simulink model "window_design"  (R2012b)
settings: Solver=ode45  StartTime=0.0  StopTime=10.0  RelTol=1e-3
undefined symbols (not defined in the file or in its folder): firceqrip, xlipgetpartsetting
libraries: xbsIndex_r4 x532, casper_library_misc x3, xps_library x2, simulink x1
(part 1 of 6)
settings Model: Creator=heystek  LastModifiedBy=heystek

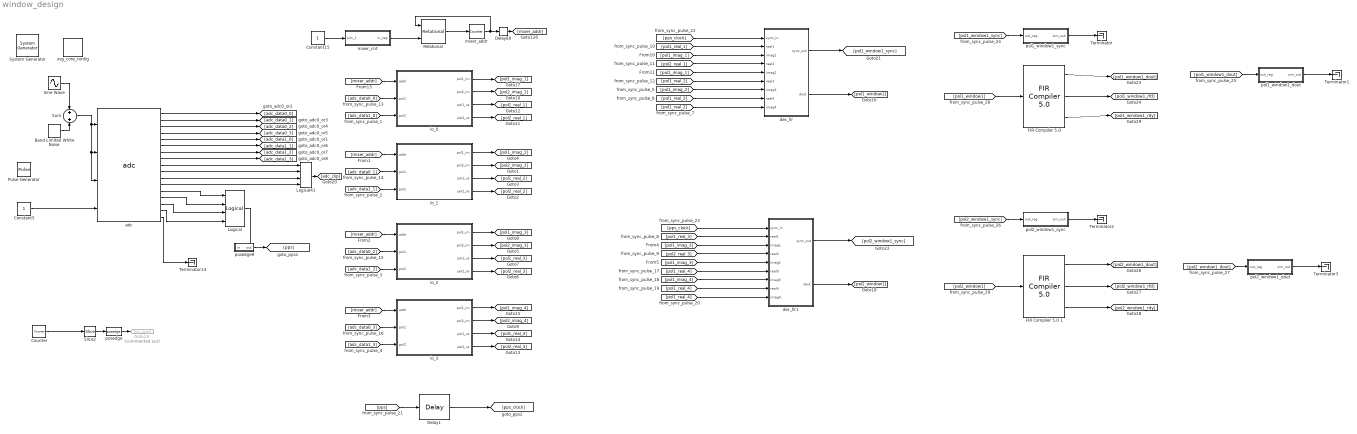
== system window_design ==
  " System Generator" : xbsIndex_r4/ System Generator  Tag=genX  xilinxfamily=virtex6  part=xc6vsx475t  speed=-1  package=ff1759  synthesis_tool=XST  clock_wrapper=Clock Enables  directory=./window_design/sysgen  proj_type=Project Navigator  Synth_file=XST Defaults  Impl_file=ISE Defaults  testbench=off  simulink_period=1  sysclk_period=6.25  dcm_input_clock_period=100  incr_netlist=off  trim_vbits=Everywhere in SubSystem  dbl_ovrd=According to Block Masks  core_generation=According to Block Masks  run_coregen=off  deprecated_control=off  eval_field=0  block_type=sysgen
  Band-Limited White Noise : simulink/Sources/Band-Limited White Noise  Cov=[0.01]  Ts=0.25  seed=[23341]
  Constant15 : Constant
  Constant5 : Constant
  Counter : xbsIndex_r4/Counter  cnt_type=Free Running  cnt_to=Inf  operation=Up  start_count=0  cnt_by_val=1  arith_type=Unsigned  n_bits=16  bin_pt=0  load_pin=off  rst=off  en=off  explicit_period=on  period=1  dbl_ovrd=off  use_behavioral_HDL=off  implementation=Fabric  block_type=counter
  Delay1 : xbsIndex_r4/Delay  rst=off  infoeditControl=Selection of Reset will increase slice count due to use of real FFs and instead of SRLs  en=off  latency=6  dbl_ovrd=off  reg_retiming=on  block_type=delay
      settings: block_version=11.4
  Delay80 : xbsIndex_r4/Delay  rst=off  infoeditControl=Selection of Reset will increase slice count due to use of real FFs and instead of SRLs  en=off  latency=2  dbl_ovrd=off  reg_retiming=on  block_type=delay
      settings: block_version=11.4
  "FIR Compiler 5.0 " : xbsIndex_r4/FIR Compiler 5.0   coefficientvector=firceqrip(5390,1e6/(800e6/2),[ 0.00057565 1e-4],'passedge')  coefficient_sets=1  filter_type=Decimation  rate_change_type=Integer  interpolation_rate=1  decimation_rate=200  zero_pack_factor=1  number_channels=1  ratespecification=Maximum_Possible  sampleperiod=1  hardwareoversamplingrate=1  filter_architecture=Systolic_Multiply_Accumulate  coefficient_reload=off  coefficient_structure=Inferred  coefficient_sign=Signed  quantization=Maximize_Dynamic_Range  coefficient_width=16  bestprecision=on  coefficient_fractional_bits=23  number_paths=1  output_rounding_mode=Convergent_Rounding_to_Even  output_width=16  allow_rounding_approximation=off  optimization_goal=Area  has_sclr=off  has_data_valid=off  has_nd=off  has_ce=off  usechan_in_adv=off  chan_in_adv=0  data_buffer_type=Automatic  coefficient_buffer_type=Automatic  input_buffer_type=Automatic  output_buffer_type=Automatic  preference_for_other_storage=Automatic  multi_column_support=Disabled  columnconfig='28'  inter_column_pipe_length=4  passband_min=0.0  passband_max=0.5  stopband_min=0.5  stopband_max=1.0  filter_selection=1  gui_behaviour=Sysgen  registered_output=true  data_sign=Signed  data_width=16  data_fractional_bits=0  wrapper_available=true  ip_wrap_arbitrary_binary_point=true  ip_name=FIR Compiler  ip_version=5.0  dsptool_ready=true  ipcore_usecache=true  ipcore_useipmodelcache=true  ipcore_xco_need_fpga_part=true  port_translation_map={ 'ce' => 'en', 'sclr' => 'rst' }  run_core_at_system_period=true  ipcore_fpga_part=xlipgetpartsetting(gcb, {'virtex4', 'xc4vsx35', '-10', 'ff668'})  structural_sim=false  block_type=fir_compiler_v5_0
  FIR Compiler 5.0 1 : xbsIndex_r4/FIR Compiler 5.0   coefficientvector=firceqrip(5390,1e6/(800e6/2),[ 0.00057565 1e-4],'passedge')  coefficient_sets=1  filter_type=Decimation  rate_change_type=Integer  interpolation_rate=1  decimation_rate=200  zero_pack_factor=1  number_channels=1  ratespecification=Maximum_Possible  sampleperiod=1  hardwareoversamplingrate=1  filter_architecture=Systolic_Multiply_Accumulate  coefficient_reload=off  coefficient_structure=Inferred  coefficient_sign=Signed  quantization=Maximize_Dynamic_Range  coefficient_width=16  bestprecision=on  coefficient_fractional_bits=23  number_paths=1  output_rounding_mode=Convergent_Rounding_to_Even  output_width=16  allow_rounding_approximation=off  optimization_goal=Area  has_sclr=off  has_data_valid=off  has_nd=off  has_ce=off  usechan_in_adv=off  chan_in_adv=0  data_buffer_type=Automatic  coefficient_buffer_type=Automatic  input_buffer_type=Automatic  output_buffer_type=Automatic  preference_for_other_storage=Automatic  multi_column_support=Disabled  columnconfig='28'  inter_column_pipe_length=4  passband_min=0.0  passband_max=0.5  stopband_min=0.5  stopband_max=1.0  filter_selection=1  gui_behaviour=Sysgen  registered_output=true  data_sign=Signed  data_width=16  data_fractional_bits=0  wrapper_available=true  ip_wrap_arbitrary_binary_point=true  ip_name=FIR Compiler  ip_version=5.0  dsptool_ready=true  ipcore_usecache=true  ipcore_useipmodelcache=true  ipcore_xco_need_fpga_part=true  port_translation_map={ 'ce' => 'en', 'sclr' => 'rst' }  run_core_at_system_period=true  ipcore_fpga_part=xlipgetpartsetting(gcb, {'virtex4', 'xc4vsx35', '-10', 'ff668'})  structural_sim=false  block_type=fir_compiler_v5_0
  Goto19 : Goto  Commented=on  GotoTag=cic_sync
  Logical : xbsIndex_r4/Logical  logical_function=OR  inputs=4  en=off  latency=0  precision=Full  arith_type=Unsigned  n_bits=16  bin_pt=0  align_bp=on  dbl_ovrd=off  block_type=logical
  Logical41 : xbsIndex_r4/Logical  logical_function=OR  inputs=4  en=off  latency=0  precision=Full  arith_type=Unsigned  n_bits=16  bin_pt=0  align_bp=on  dbl_ovrd=off  block_type=logical
  Pulse Generator : DiscretePulseGenerator  Period=800e6  PulseWidth=16  PhaseDelay=80  SampleTime=0.25
  Relational : xbsIndex_r4/Relational  mode=a=b  en=off  latency=1  dbl_ovrd=off  block_type=relational
  Sine Wave : Sin  SineType=Sample based  Amplitude=0.8  Frequency=5  Samples=2048  SampleTime=0.25  Offset=1
  Slice2 : xbsIndex_r4/Slice  nbits=1  boolean_output=on  mode=Upper Bit Location + Width  bit1=0  base1=MSB of Input  bit0=0  base0=LSB of Input  dbl_ovrd=off  block_type=slice
  Sum : Sum
  Terminator{,1..3,14} (5 alike) : Terminator
  adc : xps_library/ADCs/adc  Tag=xps:adc  adc_brd=adc0  adc_clk_rate=640  adc_interleave=off  sample_period=1
  dec_fir : Subsystem  Tag=casper:dec_fir  AncestorBlock=casper_library_downconverter/dec_fir  mask(dec_fir){n_inputs=4, coeff=[0:15], n_bits=8, n_bits_bp=7, quantization=Round  (unbiased: +/- Inf), add_latency=1, mult_latency=2, conv_latency=2, coeff_bit_width=25, coeff_bin_pt=24, absorb_adders=on, adder_imp=DSP48, lshift=1}
      mask prompts: n_inputs "Number of Parallel Streams"; coeff "Coefficients"; n_bits "Bit Width Out"; n_bits_bp "Bin Pt Out"; quantization "Quantization Behavior"; add_latency "Add Latency"; mult_latency "Mult Latency"; conv_latency "Convert latency"; coeff_bit_width "Coefficient bit width"; coeff_bin_pt "Coefficient binary point"; absorb_adders "Absorb adders into DSP slices"; adder_imp "Adder implementation"; lshift "Post adder-tree shift"
      mask help: FIR filter which can handle multiple time samples in parallel and decimates down to 1 time sample. If coefficients are symmetric, will automatically fold before multiplying.
      mask init:
      | dec_fir_init(gcb, ...
      |     'n_inputs', n_inputs, ...
      |     'coeff', coeff, ...
      |     'n_bits', n_bits, ...
      |     'n_bits_bp', n_bits_bp, ...
      |     'quantization', quantization, ...
      |     'add_latency', add_latency, ...
      |     'mult_latency', mult_latency, ...
      |     'conv_latency', conv_latency, ...
      |     'coeff_bit_width', coeff_bit_width, ...
      |     'coeff_bin_pt', coeff_bin_pt, ...
      |     'absorb_adders', absorb_adders, ...
      |     'adder_imp', adder_imp, ...
      |     'lshift', lshift);
      settings: AttributesFormatString=|
      | 16 taps
      | 8_7 r/i
      mask TypeOptions quantization: Truncate | Round  (unbiased: +/- Inf) | Round  (unbiased: Even Values)
      mask TypeOptions adder_imp: Behavioral | Fabric | DSP48
  dec_fir1 : Subsystem  Tag=casper:dec_fir  AncestorBlock=casper_library_downconverter/dec_fir  mask(dec_fir){n_inputs=4, coeff=[0:15], n_bits=8, n_bits_bp=7, quantization=Round  (unbiased: +/- Inf), add_latency=1, mult_latency=2, conv_latency=2, coeff_bit_width=25, coeff_bin_pt=24, absorb_adders=on, adder_imp=DSP48, lshift=1}
      mask prompts: n_inputs "Number of Parallel Streams"; coeff "Coefficients"; n_bits "Bit Width Out"; n_bits_bp "Bin Pt Out"; quantization "Quantization Behavior"; add_latency "Add Latency"; mult_latency "Mult Latency"; conv_latency "Convert latency"; coeff_bit_width "Coefficient bit width"; coeff_bin_pt "Coefficient binary point"; absorb_adders "Absorb adders into DSP slices"; adder_imp "Adder implementation"; lshift "Post adder-tree shift"
      mask help: FIR filter which can handle multiple time samples in parallel and decimates down to 1 time sample. If coefficients are symmetric, will automatically fold before multiplying.
      mask init: same as window_design/dec_fir
      settings: AttributesFormatString=|
      | 16 taps
      | 8_7 r/i
      mask TypeOptions quantization: Truncate | Round  (unbiased: +/- Inf) | Round  (unbiased: Even Values)
      mask TypeOptions adder_imp: Behavioral | Fabric | DSP48
  lo_0 : Subsystem  AncestorBlock=gbt_library/complex_mix_lo
  lo_1 : Subsystem  AncestorBlock=gbt_library/complex_mix_lo
  lo_2 : Subsystem  AncestorBlock=gbt_library/complex_mix_lo
  lo_3 : Subsystem  AncestorBlock=gbt_library/complex_mix_lo
  mixer_addr : xbsIndex_r4/Counter  cnt_type=Free Running  cnt_to=Inf  operation=Up  start_count=0  cnt_by_val=1  arith_type=Unsigned  n_bits=11  bin_pt=0  load_pin=off  rst=on  en=off  explicit_period=on  period=1  dbl_ovrd=off  use_behavioral_HDL=off  implementation=Fabric  block_type=counter
      settings: block_version=11.4
  mixer_cnt : Subsystem  Tag=xps:sw_reg  AncestorBlock=xps_library/software_register  mask(swreg){io_dir=From Processor, io_delay=0, sample_period=1, names=reg, bitwidths=32, bin_pts=0, arith_types=0, sim_port=on, show_format=on}
      mask prompts: io_dir "I/O direction"; io_delay "I/O delay"; sample_period "Sample period"; names "Bitfield names [msb...lsb]"; bitwidths "Bitfield widths"; bin_pts "Bitfield binary pts"; arith_types "Bitfield types, ufix=0, fix=1, bool=2"; sim_port "Provide sim input/output?"; show_format "Print format string?"
      mask help: A 32-bit software-accessible register. Can be divided into bitfields of varying widths and types using the fields in the block mask.
      mask init:
      | try
      |     swreg_init(gcb)
      | catch ex
      |     disp(sprintf('%s: %s', gcb, ex.message))
      |     errordlg(ex.message)
      | end
      settings: AttributesFormatString=1input:uf32.0 = 32 bits
      mask TypeOptions io_dir: To Processor | From Processor
      mask Callback io_dir:
      | mask_enables = get_param(gcb, 'MaskEnables');
      | mask_names = get_param(gcb, 'MaskNames');
      | if strcmp(get_param(gcb, 'io_dir'), 'To Processor'),
      |     mask_enables{ismember(mask_names, 'sample_period')} = 'off';
      | else
      |     mask_enables{ismember(mask_names, 'sample_period')} = 'on';
      | end
      | set_param(gcb, 'MaskEnables', mask_enables);
  pol1_window1_dout : Subsystem  Tag=xps:sw_reg  AncestorBlock=xps_library/software_register  mask(swreg){io_dir=To Processor, io_delay=0, sample_period=1, names=reg, bitwidths=16, bin_pts=0, arith_types=1, sim_port=on, show_format=on}
      mask prompts: io_dir "I/O direction"; io_delay "I/O delay"; sample_period "Sample period"; names "Bitfield names [msb...lsb]"; bitwidths "Bitfield widths"; bin_pts "Bitfield binary pts"; arith_types "Bitfield types, ufix=0, fix=1, bool=2"; sim_port "Provide sim input/output?"; show_format "Print format string?"
      mask help: A 32-bit software-accessible register. Can be divided into bitfields of varying widths and types using the fields in the block mask.
      mask init:
      | try
      |     swreg_init(gcb)
      | catch ex
      |     disp(sprintf('%s: %s', gcb, ex.message))
      |     errordlg(ex.message)
      | end
      settings: AttributesFormatString=1output:f16.0 = 16 bits
      mask TypeOptions io_dir: To Processor | From Processor
      mask Callback io_dir:
      | mask_enables = get_param(gcb, 'MaskEnables');
      | mask_names = get_param(gcb, 'MaskNames');
      | if strcmp(get_param(gcb, 'io_dir'), 'To Processor'),
      |     mask_enables{ismember(mask_names, 'sample_period')} = 'off';
      | else
      |     mask_enables{ismember(mask_names, 'sample_period')} = 'on';
      | end
      | set_param(gcb, 'MaskEnables', mask_enables);
  pol1_window1_sync : Subsystem  Tag=xps:sw_reg  AncestorBlock=xps_library/software_register  mask(swreg){io_dir=To Processor, io_delay=0, sample_period=1, names=reg, bitwidths=16, bin_pts=0, arith_types=2, sim_port=on, show_format=on}
      mask prompts: io_dir "I/O direction"; io_delay "I/O delay"; sample_period "Sample period"; names "Bitfield names [msb...lsb]"; bitwidths "Bitfield widths"; bin_pts "Bitfield binary pts"; arith_types "Bitfield types, ufix=0, fix=1, bool=2"; sim_port "Provide sim input/output?"; show_format "Print format string?"
      mask help: A 32-bit software-accessible register. Can be divided into bitfields of varying widths and types using the fields in the block mask.
      mask init:
      | try
      |     swreg_init(gcb)
      | catch ex
      |     disp(sprintf('%s: %s', gcb, ex.message))
      |     errordlg(ex.message)
      | end
      settings: AttributesFormatString=1output:b = 16 bits
      mask TypeOptions io_dir: To Processor | From Processor
      mask Callback io_dir:
      | mask_enables = get_param(gcb, 'MaskEnables');
      | mask_names = get_param(gcb, 'MaskNames');
      | if strcmp(get_param(gcb, 'io_dir'), 'To Processor'),
      |     mask_enables{ismember(mask_names, 'sample_period')} = 'off';
      | else
      |     mask_enables{ismember(mask_names, 'sample_period')} = 'on';
      | end
      | set_param(gcb, 'MaskEnables', mask_enables);
  pol2_window1_dout : Subsystem  Tag=xps:sw_reg  AncestorBlock=xps_library/software_register  mask(swreg){io_dir=To Processor, io_delay=0, sample_period=1, names=reg, bitwidths=16, bin_pts=0, arith_types=1, sim_port=on, show_format=on}
      mask prompts: io_dir "I/O direction"; io_delay "I/O delay"; sample_period "Sample period"; names "Bitfield names [msb...lsb]"; bitwidths "Bitfield widths"; bin_pts "Bitfield binary pts"; arith_types "Bitfield types, ufix=0, fix=1, bool=2"; sim_port "Provide sim input/output?"; show_format "Print format string?"
      mask help: A 32-bit software-accessible register. Can be divided into bitfields of varying widths and types using the fields in the block mask.
      mask init:
      | try
      |     swreg_init(gcb)
      | catch ex
      |     disp(sprintf('%s: %s', gcb, ex.message))
      |     errordlg(ex.message)
      | end
      settings: AttributesFormatString=1output:f16.0 = 16 bits
      mask TypeOptions io_dir: To Processor | From Processor
      mask Callback io_dir:
      | mask_enables = get_param(gcb, 'MaskEnables');
      | mask_names = get_param(gcb, 'MaskNames');
      | if strcmp(get_param(gcb, 'io_dir'), 'To Processor'),
      |     mask_enables{ismember(mask_names, 'sample_period')} = 'off';
      | else
      |     mask_enables{ismember(mask_names, 'sample_period')} = 'on';
      | end
      | set_param(gcb, 'MaskEnables', mask_enables);
  pol2_window1_sync : Subsystem  Tag=xps:sw_reg  AncestorBlock=xps_library/software_register  mask(swreg){io_dir=To Processor, io_delay=0, sample_period=1, names=reg, bitwidths=16, bin_pts=0, arith_types=2, sim_port=on, show_format=on}
      mask prompts: io_dir "I/O direction"; io_delay "I/O delay"; sample_period "Sample period"; names "Bitfield names [msb...lsb]"; bitwidths "Bitfield widths"; bin_pts "Bitfield binary pts"; arith_types "Bitfield types, ufix=0, fix=1, bool=2"; sim_port "Provide sim input/output?"; show_format "Print format string?"
      mask help: A 32-bit software-accessible register. Can be divided into bitfields of varying widths and types using the fields in the block mask.
      mask init:
      | try
      |     swreg_init(gcb)
      | catch ex
      |     disp(sprintf('%s: %s', gcb, ex.message))
      |     errordlg(ex.message)
      | end
      settings: AttributesFormatString=1output:b = 16 bits
      mask TypeOptions io_dir: To Processor | From Processor
      mask Callback io_dir:
      | mask_enables = get_param(gcb, 'MaskEnables');
      | mask_names = get_param(gcb, 'MaskNames');
      | if strcmp(get_param(gcb, 'io_dir'), 'To Processor'),
      |     mask_enables{ismember(mask_names, 'sample_period')} = 'off';
      | else
      |     mask_enables{ismember(mask_names, 'sample_period')} = 'on';
      | end
      | set_param(gcb, 'MaskEnables', mask_enables);
  posedge : casper_library_misc/posedge  Tag=Rising Edge Detector
  posedge9 : Subsystem  AncestorBlock=casper_library_misc/edge_detect  mask(edge_detect){edge=Rising, polarity=Active High, x_in=[0 0.08 0.08 0.16 0.16 0.24 0.24 0.32 0.32 0.4], y_in=[-1 -1  1  1  1  1  1  1  1  1], x_out=[0.6 0.68 0.68 0.76 0.76 0.84 0.84 0.92 0.92 1], y_out=[-1 -1  1  1 -1 -1 -1 -1 -1 -1]}
      mask prompts: edge "Edge Type"; polarity "Output Polarity"; x_in "Input X Positions"; y_in "Input Y Positions"; x_out "Output X Positions"; y_out "Output Y Positions"
      mask help: Output is active for one-cycle after each edge of the specified type (i.e. rising, falling or both).
      mask init:
      | edge_detect_init(gcb,...
      |     'edge',edge,...
      |     'polarity',polarity,...
      |     'x_in',x_in,...
      |     'x_out',x_out,...
      |     'y_in',y_in,...
      |     'y_out',y_out);
      | 
      | x_in_num=str2num(getfield(getfield(get_param(gcb,'UserData'),'parameters'),'x_in'));
      | x_out_num=str2num(getfield(getfield(get_param(gcb,'UserData'),'parameters'),'x_out'));
      | y_in_num=str2num(getfield(getfield(get_param(gcb,'UserData'),'parameters'),'y_in'));
      | y_out_num=str2num(getfield(getfield(get_param(gcb,'UserData'),'parameters'),'y_out'));
      settings: AttributesFormatString=|
      | rising edges
      | active high
      mask Help: Output is active for one-cycle after each edge of the specified type (i.e. rising, falling, or both).  Latency is zero.
      mask TypeOptions edge: Rising | Falling | Both
      mask TypeOptions polarity: Active High | Active Low
      mask Display:
      | plot(x_in_num,0.5+y_in_num*0.2);
      | plot(x_out_num,0.5+y_out_num*0.2);
  xsg_core_config : xps_library/XSG_core_config  Tag=xps:xsg  hw_sys=ROACH2:sx475t  clk_src=sys_clk  ROACH_clk_src=adc0_clk  ROACH2_clk_src=sys_clk  MKDIG_clk_src=sys_clk  clk_rate=160  sample_period=1  synthesis_tool=XST
  wires:
  Band-Limited White Noise/1 -> Sum/2
  Sine Wave/1 -> Sum/1
  Sum/1 -> adc/1, adc/2, adc/3
  Constant5/1 -> adc/4
  [mixer_addr] -> lo_0/1(addr)
  lo_0/1(pol1_im) -> [pol1_imag_1]
  lo_0/2(pol2_im) -> [pol2_imag_1]
  lo_0/3(pol1_re) -> [pol1_real_1]
  lo_0/4(pol2_re) -> [pol2_real_1]
  [adc_data0_0] -> lo_0/2(pol1)
  [adc_data1_0] -> lo_0/3(pol2)
  [mixer_addr] -> lo_1/1(addr)
  lo_1/1(pol1_im) -> [pol1_imag_2]
  lo_1/2(pol2_im) -> [pol2_imag_2]
  lo_1/3(pol1_re) -> [pol1_real_2]
  lo_1/4(pol2_re) -> [pol2_real_2]
  [mixer_addr] -> lo_2/1(addr)
  lo_2/1(pol1_im) -> [pol1_imag_3]
  lo_2/2(pol2_im) -> [pol2_imag_3]
  lo_2/3(pol1_re) -> [pol1_real_3]
  lo_2/4(pol2_re) -> [pol2_real_3]
  [adc_data0_1] -> lo_1/2(pol1)
  [adc_data1_1] -> lo_1/3(pol2)
  [adc_data0_2] -> lo_2/2(pol1)
  [adc_data1_2] -> lo_2/3(pol2)
  [mixer_addr] -> lo_3/1(addr)
  lo_3/1(pol1_im) -> [pol1_imag_4]
  lo_3/2(pol2_im) -> [pol2_imag_4]
  lo_3/3(pol1_re) -> [pol1_real_4]
  lo_3/4(pol2_re) -> [pol2_real_4]
  [adc_data0_3] -> lo_3/2(pol1)
  [adc_data1_3] -> lo_3/3(pol2)
  mixer_addr/1 -> Relational/1, Delay80/1
  Delay80/1 -> [mixer_addr]
  Relational/1 -> mixer_addr/1
  mixer_cnt/1(in_reg) -> Relational/2
  Constant15/1 -> mixer_cnt/1(sim_1)
  adc/1 -> [adc_data0_0]
  adc/2 -> [adc_data0_1]
  adc/3 -> [adc_data0_2]
  adc/4 -> [adc_data0_3]
  adc/5 -> [adc_data1_0]
  adc/6 -> [adc_data1_1]
  adc/7 -> [adc_data1_2]
  adc/8 -> [adc_data1_3]
  [pol1_real_1] -> dec_fir/2(real1)
  [pol1_imag_1] -> dec_fir/3(imag1)
  [pol2_real_1] -> dec_fir/4(real2)
  [pol1_imag_1] -> dec_fir/5(imag2)
  [pol1_real_2] -> dec_fir/6(real3)
  [pol1_imag_2] -> dec_fir/7(imag3)
  [pol1_real_2] -> dec_fir/8(real4)
  [pol1_real_2] -> dec_fir/9(imag4)
  [pol1_real_3] -> dec_fir1/2(real1)
  [pol1_imag_3] -> dec_fir1/3(imag1)
  [pol2_real_3] -> dec_fir1/4(real2)
  [pol1_imag_3] -> dec_fir1/5(imag2)
  [pol1_real_4] -> dec_fir1/6(real3)
  [pol1_imag_4] -> dec_fir1/7(imag3)
  [pol1_real_4] -> dec_fir1/8(real4)
  [pol1_real_4] -> dec_fir1/9(imag4)
  dec_fir/2(dout) -> [pol1_window1]
  dec_fir1/2(dout) -> [pol2_window1]
  Slice2/1 -> posedge/1
  posedge/1 -> Goto19/1
  adc/9 -> Logical41/1
  adc/10 -> Logical41/2
  adc/11 -> Logical41/3
  adc/12 -> Logical41/4
  Logical41/1 -> [adc_clip]
  adc/14 -> Logical/2
  adc/15 -> Logical/3
  adc/16 -> Logical/4
  adc/17 -> Terminator14/1
  Logical/1 -> posedge9/1(in)
  dec_fir/1(sync_out) -> [pol1_window1_sync]
  dec_fir1/1(sync_out) -> [pol2_window1_sync]
  [pps_clock] -> dec_fir/1(sync_in)
  [pps_clock] -> dec_fir1/1(sync_in)
  Counter/1 -> Slice2/1
  adc/13 -> Logical/1
  posedge9/1(out) -> [pps]
  [pps] -> Delay1/1
  Delay1/1 -> [pps_clock]
  [pol1_window1_dout] -> pol1_window1_dout/1(out_reg)
  pol1_window1_dout/1(sim_out) -> Terminator1/1
  [pol2_window1_dout] -> pol2_window1_dout/1(out_reg)
  pol2_window1_dout/1(sim_out) -> Terminator3/1
  [pol1_window1_sync] -> pol1_window1_sync/1(out_reg)
  pol1_window1_sync/1(sim_out) -> Terminator/1
  [pol2_window1_sync] -> pol2_window1_sync/1(out_reg)
  pol2_window1_sync/1(sim_out) -> Terminator2/1
  [pol1_window1] -> "FIR Compiler 5.0 "/1
  "FIR Compiler 5.0 "/1 -> [pol1_window1_dout]
  "FIR Compiler 5.0 "/2 -> [pol1_window1_rfd]
  [pol2_window1] -> FIR Compiler 5.0 1/1
  FIR Compiler 5.0 1/1 -> [pol2_window1_dout]
  FIR Compiler 5.0 1/2 -> [pol2_window1_rfd]
  FIR Compiler 5.0 1/3 -> [pol2_window1_rdy]
  "FIR Compiler 5.0 "/3 -> [pol1_window1_rdy]

== system window_design/dec_fir ==
  sync_in : Inport
  real1 : Inport  Port=2
  imag1 : Inport  Port=3
  real2 : Inport  Port=4
  imag2 : Inport  Port=5
  real3 : Inport  Port=6
  imag3 : Inport  Port=7
  real4 : Inport  Port=8
  imag4 : Inport  Port=9
  convert1 : xbsIndex_r4/Convert  gui_display_data_type=Fixed-point  arith_type="Signed  (2's comp)"  n_bits=8  bin_pt=7  float_type=Single  exp_bits=8  fraction_bits=24  quantization="Round  (unbiased: +/- Inf)"  overflow=Wrap  en=off  latency=2  dbl_ovrd=off  pipeline=off  block_type=convert
  convert2 : xbsIndex_r4/Convert  gui_display_data_type=Fixed-point  arith_type="Signed  (2's comp)"  n_bits=8  bin_pt=7  float_type=Single  exp_bits=8  fraction_bits=24  quantization="Round  (unbiased: +/- Inf)"  overflow=Wrap  en=off  latency=2  dbl_ovrd=off  pipeline=off  block_type=convert
  delay : xbsIndex_r4/Delay  rst=off  infoeditControl=Selection of Reset will increase slice count due to use of real FFs and instead of SRLs  en=off  latency=6  dbl_ovrd=off  reg_retiming=off  block_type=delay
  fir_col1 : Subsystem  AncestorBlock=casper_library_downconverter/fir_col  mask(fir_col){n_inputs=4, coeff=[3  2  1  0], add_latency=1, mult_latency=2, coeff_bit_width=25, coeff_bin_pt=24, first_stage_hdl=on, adder_imp=DSP48}
      mask prompts: n_inputs "Inputs"; coeff "Coefficients"; add_latency "Add latency"; mult_latency "Mult Latency"; coeff_bit_width "Coefficient bit width"; coeff_bin_pt "Coefficient binary point"; first_stage_hdl "Implement first stage of adder trees on output as behavioural HDL"; adder_imp "Adder implementation"
      mask init:
      | fir_col_init(gcb, ...
      |     'n_inputs', n_inputs,...
      |     'coeff', coeff, ...
      |     'mult_latency', mult_latency, ...
      |     'add_latency', add_latency, ...
      |     'coeff_bit_width', coeff_bit_width, ...
      |     'coeff_bin_pt', coeff_bin_pt, ...
      |     'first_stage_hdl', first_stage_hdl, ...
      |     'adder_imp', adder_imp);
      mask Help: eval('xlWeb(''http://casper.berkeley.edu/wiki/Fir_col'')')
      mask TypeOptions adder_imp: Behavioral | Fabric | DSP48
  fir_col2 : Subsystem  AncestorBlock=casper_library_downconverter/fir_col  mask(fir_col){n_inputs=4, coeff=[7  6  5  4], add_latency=1, mult_latency=2, coeff_bit_width=25, coeff_bin_pt=24, first_stage_hdl=on, adder_imp=DSP48}
      mask prompts: n_inputs "Inputs"; coeff "Coefficients"; add_latency "Add latency"; mult_latency "Mult Latency"; coeff_bit_width "Coefficient bit width"; coeff_bin_pt "Coefficient binary point"; first_stage_hdl "Implement first stage of adder trees on output as behavioural HDL"; adder_imp "Adder implementation"
      mask init: same as window_design/dec_fir/fir_col1
      mask Help: eval('xlWeb(''http://casper.berkeley.edu/wiki/Fir_col'')')
      mask TypeOptions adder_imp: Behavioral | Fabric | DSP48
  fir_col3 : Subsystem  AncestorBlock=casper_library_downconverter/fir_col  mask(fir_col){n_inputs=4, coeff=[11  10   9   8], add_latency=1, mult_latency=2, coeff_bit_width=25, coeff_bin_pt=24, first_stage_hdl=on, adder_imp=DSP48}
      mask prompts: n_inputs "Inputs"; coeff "Coefficients"; add_latency "Add latency"; mult_latency "Mult Latency"; coeff_bit_width "Coefficient bit width"; coeff_bin_pt "Coefficient binary point"; first_stage_hdl "Implement first stage of adder trees on output as behavioural HDL"; adder_imp "Adder implementation"
      mask init: same as window_design/dec_fir/fir_col1
      mask Help: eval('xlWeb(''http://casper.berkeley.edu/wiki/Fir_col'')')
      mask TypeOptions adder_imp: Behavioral | Fabric | DSP48
  fir_col4 : Subsystem  AncestorBlock=casper_library_downconverter/fir_col  mask(fir_col){n_inputs=4, coeff=[15  14  13  12], add_latency=1, mult_latency=2, coeff_bit_width=25, coeff_bin_pt=24, first_stage_hdl=on, adder_imp=DSP48}
      mask prompts: n_inputs "Inputs"; coeff "Coefficients"; add_latency "Add latency"; mult_latency "Mult Latency"; coeff_bit_width "Coefficient bit width"; coeff_bin_pt "Coefficient binary point"; first_stage_hdl "Implement first stage of adder trees on output as behavioural HDL"; adder_imp "Adder implementation"
      mask init: same as window_design/dec_fir/fir_col1
      mask Help: eval('xlWeb(''http://casper.berkeley.edu/wiki/Fir_col'')')
      mask TypeOptions adder_imp: Behavioral | Fabric | DSP48
  imag_sum : Subsystem  AncestorBlock=casper_library_misc/adder_tree  mask(adder_tree){n_inputs=4, latency=1, adder_imp=DSP48, first_stage_hdl=off}
      mask prompts: n_inputs "Number of Inputs"; latency "Add Latency"; adder_imp "Adder implementation"; first_stage_hdl "Use behavioural HDL for first stage of adders"
      mask help:
      | Sums all inputs using a tree of adds and delays.
      |
      | Number of inputs: The number of inputs to the block to be summed
      | Add latency: The number of clock cycles to perform one addition (affects timing)..
      | Adder implementation: choice of fabric or DSP48E core, or behavioral HDL
      | Use behavioural HDL for first stage of adders: Causes the first stage of adders to be absorbed into DSP blocks if multipliers precede them (Virtex 5). Overrides Adder implementation
      mask init:
      | adder_tree_init(gcb, ...
      |     'n_inputs', n_inputs, ...
      |     'latency', latency, ...
      |     'adder_imp', adder_imp, ...
      |     'first_stage_hdl', first_stage_hdl);
      settings: AttributesFormatString=latency 2
      mask Help: eval('xlWeb(''http://casper.berkeley.edu/wiki/Adder_tree'')')
      mask TypeOptions adder_imp: Behavioral | Fabric | DSP48
  real_sum : Subsystem  AncestorBlock=casper_library_misc/adder_tree  mask(adder_tree){n_inputs=4, latency=1, adder_imp=DSP48, first_stage_hdl=off}
      mask prompts: n_inputs "Number of Inputs"; latency "Add Latency"; adder_imp "Adder implementation"; first_stage_hdl "Use behavioural HDL for first stage of adders"
      mask help:
      | Sums all inputs using a tree of adds and delays.
      |
      | Number of inputs: The number of inputs to the block to be summed
      | Add latency: The number of clock cycles to perform one addition (affects timing)..
      | Adder implementation: choice of fabric or DSP48E core, or behavioral HDL
      | Use behavioural HDL for first stage of adders: Causes the first stage of adders to be absorbed into DSP blocks if multipliers precede them (Virtex 5). Overrides Adder implementation
      mask init:
      | adder_tree_init(gcb, ...
      |     'n_inputs', n_inputs, ...
      |     'latency', latency, ...
      |     'adder_imp', adder_imp, ...
      |     'first_stage_hdl', first_stage_hdl);
      settings: AttributesFormatString=latency 2
      mask Help: eval('xlWeb(''http://casper.berkeley.edu/wiki/Adder_tree'')')
      mask TypeOptions adder_imp: Behavioral | Fabric | DSP48
  ri_to_c : casper_library_misc/ri_to_c
  shift1 : xbsIndex_r4/Shift  shift_dir=Left  shift_bits=1  en=off  latency=0  precision=Full  arith_type="Signed  (2's comp)"  n_bits=16  bin_pt=14  quantization=Truncate  overflow=Wrap  dbl_ovrd=off  block_type=shift
  shift2 : xbsIndex_r4/Shift  shift_dir=Left  shift_bits=1  en=off  latency=0  precision=Full  arith_type="Signed  (2's comp)"  n_bits=16  bin_pt=14  quantization=Truncate  overflow=Wrap  dbl_ovrd=off  block_type=shift
  sync_out : Outport
  dout : Outport  Port=2
  wires:
  real1/1 -> fir_col1/1(real1)
  imag1/1 -> fir_col1/2(imag1)
  real2/1 -> fir_col1/3(real2)
  imag2/1 -> fir_col1/4(imag2)
  real3/1 -> fir_col1/5(real3)
  imag3/1 -> fir_col1/6(imag3)
  real4/1 -> fir_col1/7(real4)
  imag4/1 -> fir_col1/8(imag4)
  fir_col1/9(real_sum) -> real_sum/2(din1)
  fir_col1/10(imag_sum) -> imag_sum/2(din1)
  fir_col1/1(real_out1) -> fir_col2/1(real1)
  fir_col1/2(imag_out1) -> fir_col2/2(imag1)
  fir_col1/3(real_out2) -> fir_col2/3(real2)
  fir_col1/4(imag_out2) -> fir_col2/4(imag2)
  fir_col1/5(real_out3) -> fir_col2/5(real3)
  fir_col1/6(imag_out3) -> fir_col2/6(imag3)
  fir_col1/7(real_out4) -> fir_col2/7(real4)
  fir_col1/8(imag_out4) -> fir_col2/8(imag4)
  fir_col2/9(real_sum) -> real_sum/3(din2)
  fir_col2/10(imag_sum) -> imag_sum/3(din2)
  fir_col2/1(real_out1) -> fir_col3/1(real1)
  fir_col2/2(imag_out1) -> fir_col3/2(imag1)
  fir_col2/3(real_out2) -> fir_col3/3(real2)
  fir_col2/4(imag_out2) -> fir_col3/4(imag2)
  fir_col2/5(real_out3) -> fir_col3/5(real3)
  fir_col2/6(imag_out3) -> fir_col3/6(imag3)
  fir_col2/7(real_out4) -> fir_col3/7(real4)
  fir_col2/8(imag_out4) -> fir_col3/8(imag4)
  fir_col3/9(real_sum) -> real_sum/4(din3)
  fir_col3/10(imag_sum) -> imag_sum/4(din3)
  fir_col3/1(real_out1) -> fir_col4/1(real1)
  fir_col3/2(imag_out1) -> fir_col4/2(imag1)
  fir_col3/3(real_out2) -> fir_col4/3(real2)
  fir_col3/4(imag_out2) -> fir_col4/4(imag2)
  fir_col3/5(real_out3) -> fir_col4/5(real3)
  fir_col3/6(imag_out3) -> fir_col4/6(imag3)
  fir_col3/7(real_out4) -> fir_col4/7(real4)
  fir_col3/8(imag_out4) -> fir_col4/8(imag4)
  fir_col4/9(real_sum) -> real_sum/5(din4)
  fir_col4/10(imag_sum) -> imag_sum/5(din4)
  real_sum/2(dout) -> shift1/1
  imag_sum/2(dout) -> shift2/1
  shift1/1 -> convert1/1
  shift2/1 -> convert2/1
  convert1/1 -> ri_to_c/1
  convert2/1 -> ri_to_c/2
  ri_to_c/1 -> dout/1
  sync_in/1 -> delay/1
  delay/1 -> real_sum/1(sync), imag_sum/1(sync)
  real_sum/1(sync_out) -> sync_out/1

== system window_design/dec_fir1 ==
  sync_in : Inport
  real1 : Inport  Port=2
  imag1 : Inport  Port=3
  real2 : Inport  Port=4
  imag2 : Inport  Port=5
  real3 : Inport  Port=6
  imag3 : Inport  Port=7
  real4 : Inport  Port=8
  imag4 : Inport  Port=9
  convert1 : xbsIndex_r4/Convert  gui_display_data_type=Fixed-point  arith_type="Signed  (2's comp)"  n_bits=8  bin_pt=7  float_type=Single  exp_bits=8  fraction_bits=24  quantization="Round  (unbiased: +/- Inf)"  overflow=Wrap  en=off  latency=2  dbl_ovrd=off  pipeline=off  block_type=convert
  convert2 : xbsIndex_r4/Convert  gui_display_data_type=Fixed-point  arith_type="Signed  (2's comp)"  n_bits=8  bin_pt=7  float_type=Single  exp_bits=8  fraction_bits=24  quantization="Round  (unbiased: +/- Inf)"  overflow=Wrap  en=off  latency=2  dbl_ovrd=off  pipeline=off  block_type=convert
  delay : xbsIndex_r4/Delay  rst=off  infoeditControl=Selection of Reset will increase slice count due to use of real FFs and instead of SRLs  en=off  latency=6  dbl_ovrd=off  reg_retiming=off  block_type=delay
  fir_col1 : Subsystem  AncestorBlock=casper_library_downconverter/fir_col  mask(fir_col){n_inputs=4, coeff=[3  2  1  0], add_latency=1, mult_latency=2, coeff_bit_width=25, coeff_bin_pt=24, first_stage_hdl=on, adder_imp=DSP48}
      mask prompts: n_inputs "Inputs"; coeff "Coefficients"; add_latency "Add latency"; mult_latency "Mult Latency"; coeff_bit_width "Coefficient bit width"; coeff_bin_pt "Coefficient binary point"; first_stage_hdl "Implement first stage of adder trees on output as behavioural HDL"; adder_imp "Adder implementation"
      mask init: same as window_design/dec_fir/fir_col1
      mask Help: eval('xlWeb(''http://casper.berkeley.edu/wiki/Fir_col'')')
      mask TypeOptions adder_imp: Behavioral | Fabric | DSP48
  fir_col2 : Subsystem  AncestorBlock=casper_library_downconverter/fir_col  mask(fir_col){n_inputs=4, coeff=[7  6  5  4], add_latency=1, mult_latency=2, coeff_bit_width=25, coeff_bin_pt=24, first_stage_hdl=on, adder_imp=DSP48}
      mask prompts: n_inputs "Inputs"; coeff "Coefficients"; add_latency "Add latency"; mult_latency "Mult Latency"; coeff_bit_width "Coefficient bit width"; coeff_bin_pt "Coefficient binary point"; first_stage_hdl "Implement first stage of adder trees on output as behavioural HDL"; adder_imp "Adder implementation"
      mask init: same as window_design/dec_fir/fir_col1
      mask Help: eval('xlWeb(''http://casper.berkeley.edu/wiki/Fir_col'')')
      mask TypeOptions adder_imp: Behavioral | Fabric | DSP48
  fir_col3 : Subsystem  AncestorBlock=casper_library_downconverter/fir_col  mask(fir_col){n_inputs=4, coeff=[11  10   9   8], add_latency=1, mult_latency=2, coeff_bit_width=25, coeff_bin_pt=24, first_stage_hdl=on, adder_imp=DSP48}
      mask prompts: n_inputs "Inputs"; coeff "Coefficients"; add_latency "Add latency"; mult_latency "Mult Latency"; coeff_bit_width "Coefficient bit width"; coeff_bin_pt "Coefficient binary point"; first_stage_hdl "Implement first stage of adder trees on output as behavioural HDL"; adder_imp "Adder implementation"
      mask init: same as window_design/dec_fir/fir_col1
      mask Help: eval('xlWeb(''http://casper.berkeley.edu/wiki/Fir_col'')')
      mask TypeOptions adder_imp: Behavioral | Fabric | DSP48
  fir_col4 : Subsystem  AncestorBlock=casper_library_downconverter/fir_col  mask(fir_col){n_inputs=4, coeff=[15  14  13  12], add_latency=1, mult_latency=2, coeff_bit_width=25, coeff_bin_pt=24, first_stage_hdl=on, adder_imp=DSP48}
      mask prompts: n_inputs "Inputs"; coeff "Coefficients"; add_latency "Add latency"; mult_latency "Mult Latency"; coeff_bit_width "Coefficient bit width"; coeff_bin_pt "Coefficient binary point"; first_stage_hdl "Implement first stage of adder trees on output as behavioural HDL"; adder_imp "Adder implementation"
      mask init: same as window_design/dec_fir/fir_col1
      mask Help: eval('xlWeb(''http://casper.berkeley.edu/wiki/Fir_col'')')
      mask TypeOptions adder_imp: Behavioral | Fabric | DSP48
  imag_sum : Subsystem  AncestorBlock=casper_library_misc/adder_tree  mask(adder_tree){n_inputs=4, latency=1, adder_imp=DSP48, first_stage_hdl=off}
      mask prompts: n_inputs "Number of Inputs"; latency "Add Latency"; adder_imp "Adder implementation"; first_stage_hdl "Use behavioural HDL for first stage of adders"
      mask help:
      | Sums all inputs using a tree of adds and delays.
      |
      | Number of inputs: The number of inputs to the block to be summed
      | Add latency: The number of clock cycles to perform one addition (affects timing)..
      | Adder implementation: choice of fabric or DSP48E core, or behavioral HDL
      | Use behavioural HDL for first stage of adders: Causes the first stage of adders to be absorbed into DSP blocks if multipliers precede them (Virtex 5). Overrides Adder implementation
      mask init:
      | adder_tree_init(gcb, ...
      |     'n_inputs', n_inputs, ...
      |     'latency', latency, ...
      |     'adder_imp', adder_imp, ...
      |     'first_stage_hdl', first_stage_hdl);
      settings: AttributesFormatString=latency 2
      mask Help: eval('xlWeb(''http://casper.berkeley.edu/wiki/Adder_tree'')')
      mask TypeOptions adder_imp: Behavioral | Fabric | DSP48
  real_sum : Subsystem  AncestorBlock=casper_library_misc/adder_tree  mask(adder_tree){n_inputs=4, latency=1, adder_imp=DSP48, first_stage_hdl=off}
      mask prompts: n_inputs "Number of Inputs"; latency "Add Latency"; adder_imp "Adder implementation"; first_stage_hdl "Use behavioural HDL for first stage of adders"
      mask help:
      | Sums all inputs using a tree of adds and delays.
      |
      | Number of inputs: The number of inputs to the block to be summed
      | Add latency: The number of clock cycles to perform one addition (affects timing)..
      | Adder implementation: choice of fabric or DSP48E core, or behavioral HDL
      | Use behavioural HDL for first stage of adders: Causes the first stage of adders to be absorbed into DSP blocks if multipliers precede them (Virtex 5). Overrides Adder implementation
      mask init:
      | adder_tree_init(gcb, ...
      |     'n_inputs', n_inputs, ...
      |     'latency', latency, ...
      |     'adder_imp', adder_imp, ...
      |     'first_stage_hdl', first_stage_hdl);
      settings: AttributesFormatString=latency 2
      mask Help: eval('xlWeb(''http://casper.berkeley.edu/wiki/Adder_tree'')')
      mask TypeOptions adder_imp: Behavioral | Fabric | DSP48
  ri_to_c : casper_library_misc/ri_to_c
  shift1 : xbsIndex_r4/Shift  shift_dir=Left  shift_bits=1  en=off  latency=0  precision=Full  arith_type="Signed  (2's comp)"  n_bits=16  bin_pt=14  quantization=Truncate  overflow=Wrap  dbl_ovrd=off  block_type=shift
  shift2 : xbsIndex_r4/Shift  shift_dir=Left  shift_bits=1  en=off  latency=0  precision=Full  arith_type="Signed  (2's comp)"  n_bits=16  bin_pt=14  quantization=Truncate  overflow=Wrap  dbl_ovrd=off  block_type=shift
  sync_out : Outport
  dout : Outport  Port=2
  wires:
  real1/1 -> fir_col1/1(real1)
  imag1/1 -> fir_col1/2(imag1)
  real2/1 -> fir_col1/3(real2)
  imag2/1 -> fir_col1/4(imag2)
  real3/1 -> fir_col1/5(real3)
  imag3/1 -> fir_col1/6(imag3)
  real4/1 -> fir_col1/7(real4)
  imag4/1 -> fir_col1/8(imag4)
  fir_col1/9(real_sum) -> real_sum/2(din1)
  fir_col1/10(imag_sum) -> imag_sum/2(din1)
  fir_col1/1(real_out1) -> fir_col2/1(real1)
  fir_col1/2(imag_out1) -> fir_col2/2(imag1)
  fir_col1/3(real_out2) -> fir_col2/3(real2)
  fir_col1/4(imag_out2) -> fir_col2/4(imag2)
  fir_col1/5(real_out3) -> fir_col2/5(real3)
  fir_col1/6(imag_out3) -> fir_col2/6(imag3)
  fir_col1/7(real_out4) -> fir_col2/7(real4)
  fir_col1/8(imag_out4) -> fir_col2/8(imag4)
  fir_col2/9(real_sum) -> real_sum/3(din2)
  fir_col2/10(imag_sum) -> imag_sum/3(din2)
  fir_col2/1(real_out1) -> fir_col3/1(real1)
  fir_col2/2(imag_out1) -> fir_col3/2(imag1)
  fir_col2/3(real_out2) -> fir_col3/3(real2)
  fir_col2/4(imag_out2) -> fir_col3/4(imag2)
  fir_col2/5(real_out3) -> fir_col3/5(real3)
  fir_col2/6(imag_out3) -> fir_col3/6(imag3)
  fir_col2/7(real_out4) -> fir_col3/7(real4)
  fir_col2/8(imag_out4) -> fir_col3/8(imag4)
  fir_col3/9(real_sum) -> real_sum/4(din3)
  fir_col3/10(imag_sum) -> imag_sum/4(din3)
  fir_col3/1(real_out1) -> fir_col4/1(real1)
  fir_col3/2(imag_out1) -> fir_col4/2(imag1)
  fir_col3/3(real_out2) -> fir_col4/3(real2)
  fir_col3/4(imag_out2) -> fir_col4/4(imag2)
  fir_col3/5(real_out3) -> fir_col4/5(real3)
  fir_col3/6(imag_out3) -> fir_col4/6(imag3)
  fir_col3/7(real_out4) -> fir_col4/7(real4)
  fir_col3/8(imag_out4) -> fir_col4/8(imag4)
  fir_col4/9(real_sum) -> real_sum/5(din4)
  fir_col4/10(imag_sum) -> imag_sum/5(din4)
  real_sum/2(dout) -> shift1/1
  imag_sum/2(dout) -> shift2/1
  shift1/1 -> convert1/1
  shift2/1 -> convert2/1
  convert1/1 -> ri_to_c/1
  convert2/1 -> ri_to_c/2
  ri_to_c/1 -> dout/1
  sync_in/1 -> delay/1
  delay/1 -> real_sum/1(sync), imag_sum/1(sync)
  real_sum/1(sync_out) -> sync_out/1

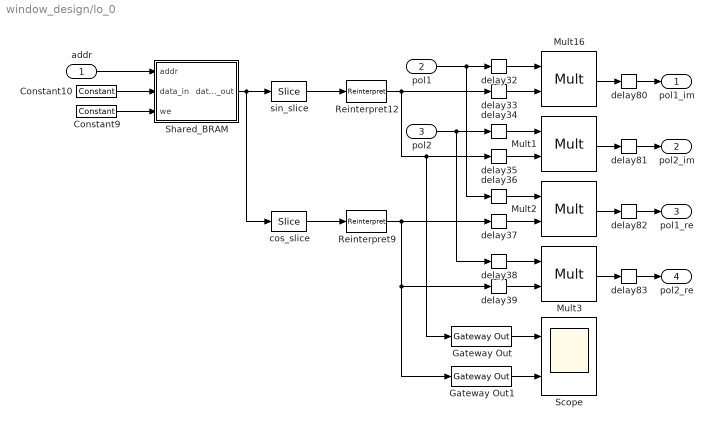
== system window_design/lo_0 ==
  addr : Inport
  pol1 : Inport  Port=2
  pol2 : Inport  Port=3
  Constant10 : xbsIndex_r4/Constant  const=0  gui_display_data_type=Fixed-point  arith_type=Unsigned  n_bits=18  bin_pt=0  preci_type=Single  exp_width=8  frac_width=24  explicit_period=on  period=1  equ=P=C  opselect=C  inp2=PCIN>>17  opr=+  inp1=P  carry=CIN  dbl_ovrd=off  block_type=constant
  Constant9 : xbsIndex_r4/Constant  const=0  gui_display_data_type=Fixed-point  arith_type=Unsigned  n_bits=18  bin_pt=0  preci_type=Single  exp_width=8  frac_width=24  explicit_period=on  period=1  equ=P=C  opselect=C  inp2=PCIN>>17  opr=+  inp1=P  carry=CIN  dbl_ovrd=off  block_type=constant
  Gateway Out : xbsIndex_r4/Gateway Out  inherit_from_input=off  hdl_port=on  timing_constraint=None  locs_specified=off  LOCs={}  UseAsDAC=off  DACChannel='1'  block_type=gatewayout
      settings: infoedit="Gateway out block.  Converts Xilinx fixed point or floating-point type inputs into ouputs of type Simulink integer, double, or fixed point.<br><br>Hardware notes:  In hardware these blocks become top level output ports or are discarded, depending on how they are configured."
  Gateway Out1 : xbsIndex_r4/Gateway Out  inherit_from_input=off  hdl_port=on  timing_constraint=None  locs_specified=off  LOCs={}  UseAsDAC=off  DACChannel='1'  block_type=gatewayout
      settings: infoedit="Gateway out block.  Converts Xilinx fixed point or floating-point type inputs into ouputs of type Simulink integer, double, or fixed point.<br><br>Hardware notes:  In hardware these blocks become top level output ports or are discarded, depending on how they are configured."
  Mult{1..3,16} (4 alike) : xbsIndex_r4/Mult  precision=User Defined  arith_type="Signed  (2's comp)"  n_bits=16  bin_pt=15  quantization=Truncate  overflow=Wrap  en=off  latency=5  dbl_ovrd=off  use_behavioral_HDL=off  opt=Speed  use_embedded=on  optimum_pipeline=off  pipeline=on  use_rpm=on  placement_style=Triangular  block_type=mult
      settings: block_version=11.4
  Reinterpret12 : xbsIndex_r4/Reinterpret  force_arith_type=on  arith_type="Signed  (2's comp)"  force_bin_pt=on  bin_pt=15  block_type=reinterpret
  Reinterpret9 : xbsIndex_r4/Reinterpret  force_arith_type=on  arith_type="Signed  (2's comp)"  force_bin_pt=on  bin_pt=15  block_type=reinterpret
      settings: infoedit="Changes signal type without altering the binary representation.   You can changed the signal between signed and unsigned, and relocate the binary point.<br><br>Hardware notes: In hardware this block costs nothing.<br><br>Example:  Suppose the input is 6 bits wide, signed, with 2 fractional bits, and the output is forced to unsigned with 0 fractional bits.  Then an input of -2.0 (1110.00 in binary 2's complement) becomes an output of 56 (111000 in binary)."
  Scope : Scope  NumInputPorts=2
      settings: YMin=-0.0075~-1  YMax=0.0075~1  SaveName=ScopeData3
  Shared_BRAM : Subsystem  Tag=xps:bram  AncestorBlock=xps_library/Shared_BRAM  mask{arith_type=Signed  (2's comp), addr_width=10, data_width=32, reg_prim_output=off, reg_core_output=off, optimization=Minimum_Area, data_bin_pt=0, init_vals=[1:2^11], sample_rate=1}
      mask prompts: arith_type "Output Data Type"; addr_width "Address width"; data_width "Data Width"; reg_prim_output "Register Primitive Output"; reg_core_output "Register Core Output"; data_bin_pt "Data Binary Point"; init_vals "Initial values (simulation only)"; sample_rate "Sample rate"
      mask init:
      | shared_bram_mask;
      mask TypeOptions arith_type: Unsigned | Signed  (2's comp)
      mask TypeOptions data_width: 8 | 16 | 32 | 64 | 128
      mask TypeOptions optimization: Minimum_Area | Low_Power
  cos_slice : xbsIndex_r4/Slice  nbits=16  boolean_output=off  mode=Lower Bit Location + Width  bit1=0  base1=MSB of Input  bit0=0  base0=LSB of Input  dbl_ovrd=off  block_type=slice
  delay{32..39,80..83} (12 alike) : xbsIndex_r4/Delay  rst=off  infoeditControl=Selection of Reset will increase slice count due to use of real FFs and instead of SRLs  en=off  latency=1  dbl_ovrd=off  reg_retiming=on  block_type=delay
      settings: block_version=11.4
  sin_slice : xbsIndex_r4/Slice  nbits=16  boolean_output=off  mode=Upper Bit Location + Width  bit1=0  base1=MSB of Input  bit0=0  base0=LSB of Input  dbl_ovrd=off  block_type=slice
  pol1_im : Outport
  pol2_im : Outport  Port=2
  pol1_re : Outport  Port=3
  pol2_re : Outport  Port=4
  wires:
  Constant9/1 -> Shared_BRAM/3(we)
  Constant10/1 -> Shared_BRAM/2(data_in)
  Mult16/1 -> delay80/1
  Reinterpret12/1 -> delay33/1, delay35/1, Gateway Out/1
  sin_slice/1 -> Reinterpret12/1
  Shared_BRAM/1(data_out) -> cos_slice/1, sin_slice/1
  Mult1/1 -> delay81/1
  Mult2/1 -> delay82/1
  Reinterpret9/1 -> delay37/1, delay39/1, Gateway Out1/1
  cos_slice/1 -> Reinterpret9/1
  Mult3/1 -> delay83/1
  delay32/1 -> Mult16/1
  delay33/1 -> Mult16/2
  delay34/1 -> Mult1/1
  delay35/1 -> Mult1/2
  delay36/1 -> Mult2/1
  delay37/1 -> Mult2/2
  delay38/1 -> Mult3/1
  delay39/1 -> Mult3/2
  delay80/1 -> pol1_im/1
  pol2/1 -> delay34/1, delay38/1
  delay81/1 -> pol2_im/1
  delay82/1 -> pol1_re/1
  delay83/1 -> pol2_re/1
  pol1/1 -> delay32/1, delay36/1
  addr/1 -> Shared_BRAM/1(addr)
  Gateway Out/1 -> Scope/1
  Gateway Out1/1 -> Scope/2
